simulink model "sampleModel7126_pp_1_1"  (R2018a)
settings: Solver=VariableStepAuto  StartTime=0.0  StopTime=10.0  RelTol=1e-3
undefined symbols (not defined in the file): DiscIntNeverNeededParam
libraries: simulink x367
(part 6 of 12)

== system sampleModel7126_pp_1_1/cfblk4 ==
  emi_839 : Inport
  Action Port : ActionPort  ActionType=then
  cfblk4 : simulink/Continuous/PID Controller  Controller=PID  TimeDomain=Discrete-time  SampleTime=1  IntegratorMethod=Forward Euler  FilterMethod=Forward Euler  Form=Parallel  UseFilter=on  ControllerParametersSource=internal  P=1  I=1  D=0  N=100  InitialConditionSource=internal  InitialConditionForIntegrator=0  InitialConditionForFilter=0  ExternalReset=none  LimitOutput=off  UpperSaturationLimit=inf  LowerSaturationLimit=-inf  LinearizeAsGain=off  AntiWindupMode=none  Kb=1  TrackingMode=off  Kt=1  PParamMin=[]  PParamMax=[]  IParamMin=[]  IParamMax=[]  DParamMin=[]  DParamMax=[]  NParamMin=[]  NParamMax=[]  KbParamMin=[]  KbParamMax=[]  KtParamMin=[]  KtParamMax=[]  POutMin=[]  POutMax=[]  IOutMin=[]  IOutMax=[]  DOutMin=[]  DOutMax=[]  NOutMin=[]  NOutMax=[]  KbOutMin=[]  KbOutMax=[]  KtOutMin=[]  KtOutMax=[]  IntegratorOutMin=[]  IntegratorOutMax=[]  FilterOutMin=[]  FilterOutMax=[]  SumOutMin=[]  SumOutMax=[]  SumI1OutMin=[]  SumI1OutMax=[]  SumI2OutMin=[]  SumI2OutMax=[]  SumI3OutMin=[]  SumI3OutMax=[]  SumDOutMin=[]  SumDOutMax=[]  SaturationOutMin=[]  SaturationOutMax=[]  IntegratorContinuousStateAttributes=''  IntegratorStateMustResolveToSignalObject=off  IntegratorRTWStateStorageClass=Auto  FilterContinuousStateAttributes=''  FilterStateMustResolveToSignalObject=off  FilterRTWStateStorageClass=Auto  DifferentiatorICPrevScaledInput=0  DifferentiatorOutMin=[]  DifferentiatorOutMax=[]  FilterDiffOutCoefMin=[]  FilterDiffOutCoefMax=[]  SumDenOutMin=[]  SumDenOutMax=[]  SumNumOutMin=[]  SumNumOutMax=[]  ReciprocalOutMin=[]  ReciprocalOutMax=[]  DivideOutMin=[]  DivideOutMax=[]  TunerSelectOption=Transfer Function Based (PID Tuner App)
  emi_840 : Outport
  wires:
  emi_839/1 -> cfblk4/1
  cfblk4/1 -> emi_840/1

== system sampleModel7126_pp_1_1/cfblk43 ==
  emi_1604 : Inport
  Action Port : ActionPort  ActionType=then
  cfblk43 : DiscreteFilter  SampleTime=1
  emi_1605 : Outport
  wires:
  emi_1604/1 -> cfblk43/1
  cfblk43/1 -> emi_1605/1

== system sampleModel7126_pp_1_1/cfblk44 ==
  emi_1231 : Inport
  emi_1232 : Inport  Port=2
  Action Port : ActionPort  ActionType=then
  cfblk44 : simulink/Continuous/PID Controller (2DOF)  Controller=PID  TimeDomain=Discrete-time  SampleTime=1  IntegratorMethod=Forward Euler  FilterMethod=Forward Euler  Form=Parallel  UseFilter=on  ControllerParametersSource=internal  P=1  I=1  D=0  N=100  b=1  c=1  InitialConditionSource=internal  InitialConditionForIntegrator=0  InitialConditionForFilter=0  ExternalReset=none  LimitOutput=off  UpperSaturationLimit=inf  LowerSaturationLimit=-inf  LinearizeAsGain=off  AntiWindupMode=none  Kb=1  TrackingMode=off  Kt=1  PParamMin=[]  PParamMax=[]  IParamMin=[]  IParamMax=[]  DParamMin=[]  DParamMax=[]  NParamMin=[]  NParamMax=[]  bParamMin=[]  bParamMax=[]  cParamMin=[]  cParamMax=[]  KbParamMin=[]  KbParamMax=[]  KtParamMin=[]  KtParamMax=[]  POutMin=[]  POutMax=[]  IOutMin=[]  IOutMax=[]  DOutMin=[]  DOutMax=[]  NOutMin=[]  NOutMax=[]  bOutMin=[]  bOutMax=[]  cOutMin=[]  cOutMax=[]  KbOutMin=[]  KbOutMax=[]  KtOutMin=[]  KtOutMax=[]  IntegratorOutMin=[]  IntegratorOutMax=[]  FilterOutMin=[]  FilterOutMax=[]  SumOutMin=[]  SumOutMax=[]  Sum1OutMin=[]  Sum1OutMax=[]  Sum2OutMin=[]  Sum2OutMax=[]  Sum3OutMin=[]  Sum3OutMax=[]  SumI1OutMin=[]  SumI1OutMax=[]  SumI2OutMin=[]  SumI2OutMax=[]  SumI3OutMin=[]  SumI3OutMax=[]  SumDOutMin=[]  SumDOutMax=[]  SaturationOutMin=[]  SaturationOutMax=[]  IntegratorContinuousStateAttributes=''  IntegratorStateMustResolveToSignalObject=off  IntegratorRTWStateStorageClass=Auto  FilterContinuousStateAttributes=''  FilterStateMustResolveToSignalObject=off  FilterRTWStateStorageClass=Auto  DifferentiatorICPrevScaledInput=0  DifferentiatorOutMin=[]  DifferentiatorOutMax=[]  FilterDiffOutCoefMin=[]  FilterDiffOutCoefMax=[]  SumDenOutMin=[]  SumDenOutMax=[]  SumNumOutMin=[]  SumNumOutMax=[]  ReciprocalOutMin=[]  ReciprocalOutMax=[]  DivideOutMin=[]  DivideOutMax=[]  TunerSelectOption=Transfer Function Based (PID Tuner App)
  emi_1233 : Outport
  wires:
  emi_1231/1 -> cfblk44/1
  emi_1232/1 -> cfblk44/2
  cfblk44/1 -> emi_1233/1

== system sampleModel7126_pp_1_1/cfblk48 ==
  emi_1269 : Inport
  Action Port : ActionPort  ActionType=then
  cfblk48 : DiscreteFir  SampleTime=1
  emi_1270 : Outport
  wires:
  emi_1269/1 -> cfblk48/1
  cfblk48/1 -> emi_1270/1

== system sampleModel7126_pp_1_1/cfblk5 ==
  emi_1928 : Inport
  Action Port : ActionPort  ActionType=then
  cfblk5 : DiscreteTransferFcn  SampleTime=1
  emi_1929 : Outport
  wires:
  emi_1928/1 -> cfblk5/1
  cfblk5/1 -> emi_1929/1

== system sampleModel7126_pp_1_1/cfblk54 ==
  emi_1166 : Inport
  Action Port : ActionPort  ActionType=then
  cfblk54 : simulink/Continuous/PID Controller  Controller=PID  TimeDomain=Discrete-time  SampleTime=1  IntegratorMethod=Forward Euler  FilterMethod=Forward Euler  Form=Parallel  UseFilter=on  ControllerParametersSource=internal  P=1  I=1  D=0  N=100  InitialConditionSource=internal  InitialConditionForIntegrator=0  InitialConditionForFilter=0  ExternalReset=none  LimitOutput=off  UpperSaturationLimit=inf  LowerSaturationLimit=-inf  LinearizeAsGain=off  AntiWindupMode=none  Kb=1  TrackingMode=off  Kt=1  PParamMin=[]  PParamMax=[]  IParamMin=[]  IParamMax=[]  DParamMin=[]  DParamMax=[]  NParamMin=[]  NParamMax=[]  KbParamMin=[]  KbParamMax=[]  KtParamMin=[]  KtParamMax=[]  POutMin=[]  POutMax=[]  IOutMin=[]  IOutMax=[]  DOutMin=[]  DOutMax=[]  NOutMin=[]  NOutMax=[]  KbOutMin=[]  KbOutMax=[]  KtOutMin=[]  KtOutMax=[]  IntegratorOutMin=[]  IntegratorOutMax=[]  FilterOutMin=[]  FilterOutMax=[]  SumOutMin=[]  SumOutMax=[]  SumI1OutMin=[]  SumI1OutMax=[]  SumI2OutMin=[]  SumI2OutMax=[]  SumI3OutMin=[]  SumI3OutMax=[]  SumDOutMin=[]  SumDOutMax=[]  SaturationOutMin=[]  SaturationOutMax=[]  IntegratorContinuousStateAttributes=''  IntegratorStateMustResolveToSignalObject=off  IntegratorRTWStateStorageClass=Auto  FilterContinuousStateAttributes=''  FilterStateMustResolveToSignalObject=off  FilterRTWStateStorageClass=Auto  DifferentiatorICPrevScaledInput=0  DifferentiatorOutMin=[]  DifferentiatorOutMax=[]  FilterDiffOutCoefMin=[]  FilterDiffOutCoefMax=[]  SumDenOutMin=[]  SumDenOutMax=[]  SumNumOutMin=[]  SumNumOutMax=[]  ReciprocalOutMin=[]  ReciprocalOutMax=[]  DivideOutMin=[]  DivideOutMax=[]  TunerSelectOption=Transfer Function Based (PID Tuner App)
  emi_1167 : Outport
  wires:
  emi_1166/1 -> cfblk54/1
  cfblk54/1 -> emi_1167/1

== system sampleModel7126_pp_1_1/cfblk57 ==
  emi_896 : Inport
  Action Port : ActionPort  ActionType=then
  cfblk57 : simulink/Continuous/PID Controller  Controller=PID  TimeDomain=Discrete-time  SampleTime=1  IntegratorMethod=Forward Euler  FilterMethod=Forward Euler  Form=Parallel  UseFilter=on  ControllerParametersSource=internal  P=1  I=1  D=0  N=100  InitialConditionSource=internal  InitialConditionForIntegrator=0  InitialConditionForFilter=0  ExternalReset=none  LimitOutput=off  UpperSaturationLimit=inf  LowerSaturationLimit=-inf  LinearizeAsGain=off  AntiWindupMode=none  Kb=1  TrackingMode=off  Kt=1  PParamMin=[]  PParamMax=[]  IParamMin=[]  IParamMax=[]  DParamMin=[]  DParamMax=[]  NParamMin=[]  NParamMax=[]  KbParamMin=[]  KbParamMax=[]  KtParamMin=[]  KtParamMax=[]  POutMin=[]  POutMax=[]  IOutMin=[]  IOutMax=[]  DOutMin=[]  DOutMax=[]  NOutMin=[]  NOutMax=[]  KbOutMin=[]  KbOutMax=[]  KtOutMin=[]  KtOutMax=[]  IntegratorOutMin=[]  IntegratorOutMax=[]  FilterOutMin=[]  FilterOutMax=[]  SumOutMin=[]  SumOutMax=[]  SumI1OutMin=[]  SumI1OutMax=[]  SumI2OutMin=[]  SumI2OutMax=[]  SumI3OutMin=[]  SumI3OutMax=[]  SumDOutMin=[]  SumDOutMax=[]  SaturationOutMin=[]  SaturationOutMax=[]  IntegratorContinuousStateAttributes=''  IntegratorStateMustResolveToSignalObject=off  IntegratorRTWStateStorageClass=Auto  FilterContinuousStateAttributes=''  FilterStateMustResolveToSignalObject=off  FilterRTWStateStorageClass=Auto  DifferentiatorICPrevScaledInput=0  DifferentiatorOutMin=[]  DifferentiatorOutMax=[]  FilterDiffOutCoefMin=[]  FilterDiffOutCoefMax=[]  SumDenOutMin=[]  SumDenOutMax=[]  SumNumOutMin=[]  SumNumOutMax=[]  ReciprocalOutMin=[]  ReciprocalOutMax=[]  DivideOutMin=[]  DivideOutMax=[]  TunerSelectOption=Transfer Function Based (PID Tuner App)
  emi_897 : Outport
  wires:
  emi_896/1 -> cfblk57/1
  cfblk57/1 -> emi_897/1

== system sampleModel7126_pp_1_1/cfblk60 ==
  emi_94 : Inport
  emi_95 : Inport  Port=2
  Action Port : ActionPort  ActionType=then
  cfblk60 : simulink/Continuous/PID Controller (2DOF)  Controller=PID  TimeDomain=Discrete-time  SampleTime=1  IntegratorMethod=Forward Euler  FilterMethod=Forward Euler  Form=Parallel  UseFilter=on  ControllerParametersSource=internal  P=1  I=1  D=0  N=100  b=1  c=1  InitialConditionSource=internal  InitialConditionForIntegrator=0  InitialConditionForFilter=0  ExternalReset=none  LimitOutput=off  UpperSaturationLimit=inf  LowerSaturationLimit=-inf  LinearizeAsGain=off  AntiWindupMode=none  Kb=1  TrackingMode=off  Kt=1  PParamMin=[]  PParamMax=[]  IParamMin=[]  IParamMax=[]  DParamMin=[]  DParamMax=[]  NParamMin=[]  NParamMax=[]  bParamMin=[]  bParamMax=[]  cParamMin=[]  cParamMax=[]  KbParamMin=[]  KbParamMax=[]  KtParamMin=[]  KtParamMax=[]  POutMin=[]  POutMax=[]  IOutMin=[]  IOutMax=[]  DOutMin=[]  DOutMax=[]  NOutMin=[]  NOutMax=[]  bOutMin=[]  bOutMax=[]  cOutMin=[]  cOutMax=[]  KbOutMin=[]  KbOutMax=[]  KtOutMin=[]  KtOutMax=[]  IntegratorOutMin=[]  IntegratorOutMax=[]  FilterOutMin=[]  FilterOutMax=[]  SumOutMin=[]  SumOutMax=[]  Sum1OutMin=[]  Sum1OutMax=[]  Sum2OutMin=[]  Sum2OutMax=[]  Sum3OutMin=[]  Sum3OutMax=[]  SumI1OutMin=[]  SumI1OutMax=[]  SumI2OutMin=[]  SumI2OutMax=[]  SumI3OutMin=[]  SumI3OutMax=[]  SumDOutMin=[]  SumDOutMax=[]  SaturationOutMin=[]  SaturationOutMax=[]  IntegratorContinuousStateAttributes=''  IntegratorStateMustResolveToSignalObject=off  IntegratorRTWStateStorageClass=Auto  FilterContinuousStateAttributes=''  FilterStateMustResolveToSignalObject=off  FilterRTWStateStorageClass=Auto  DifferentiatorICPrevScaledInput=0  DifferentiatorOutMin=[]  DifferentiatorOutMax=[]  FilterDiffOutCoefMin=[]  FilterDiffOutCoefMax=[]  SumDenOutMin=[]  SumDenOutMax=[]  SumNumOutMin=[]  SumNumOutMax=[]  ReciprocalOutMin=[]  ReciprocalOutMax=[]  DivideOutMin=[]  DivideOutMax=[]  TunerSelectOption=Transfer Function Based (PID Tuner App)
  emi_96 : Outport
  wires:
  emi_94/1 -> cfblk60/1
  emi_95/1 -> cfblk60/2
  cfblk60/1 -> emi_96/1

== system sampleModel7126_pp_1_1/cfblk61 ==
  emi_1138 : Inport
  Action Port : ActionPort  ActionType=then
  cfblk61 : UnitDelay
  emi_1139 : Outport
  wires:
  emi_1138/1 -> cfblk61/1
  cfblk61/1 -> emi_1139/1

== system sampleModel7126_pp_1_1/cfblk67 ==
  emi_437 : Inport
  emi_438 : Inport  Port=2
  Action Port : ActionPort  ActionType=then
  cfblk67 : Delay  ShowEnablePort=on  SampleTime=1
      settings: InputPortMap=u0,e6
  emi_439 : Outport
  wires:
  emi_437/1 -> cfblk67/1
  emi_438/1 -> cfblk67/2
  cfblk67/1 -> emi_439/1

== system sampleModel7126_pp_1_1/cfblk7 ==
  emi_1540 : Inport
  Action Port : ActionPort  ActionType=then
  cfblk7 : UnitDelay
  emi_1541 : Outport
  wires:
  emi_1540/1 -> cfblk7/1
  cfblk7/1 -> emi_1541/1

== system sampleModel7126_pp_1_1/cfblk74 ==
  emi_1569 : Inport
  Action Port : ActionPort  ActionType=then
  cfblk74 : simulink/Discrete/Tapped Delay  vinit=0.0  samptime=-1  NumDelays=1  DelayOrder=Oldest  includeCurrent=off
  emi_1570 : Outport
  wires:
  emi_1569/1 -> cfblk74/1
  cfblk74/1 -> emi_1570/1

== system sampleModel7126_pp_1_1/cfblk82 ==
  emi_2052 : Inport
  Action Port : ActionPort  ActionType=then
  cfblk82 : DiscreteTransferFcn  SampleTime=1
  emi_2053 : Outport
  wires:
  emi_2052/1 -> cfblk82/1
  cfblk82/1 -> emi_2053/1

== system sampleModel7126_pp_1_1/cfblk84 ==
  emi_2166 : Inport
  Action Port : ActionPort  ActionType=then
  cfblk84 : UnitDelay
  emi_2167 : Outport
  wires:
  emi_2166/1 -> cfblk84/1
  cfblk84/1 -> emi_2167/1

== system sampleModel7126_pp_1_1/cfblk85 ==
  emi_15 : Inport
  Action Port : ActionPort  ActionType=then
  cfblk85 : DiscreteStateSpace
  emi_16 : Outport
  wires:
  emi_15/1 -> cfblk85/1
  cfblk85/1 -> emi_16/1

== system sampleModel7126_pp_1_1/cfblk9 ==
  emi_365 : Inport
  Action Port : ActionPort  ActionType=then
  cfblk9 : DiscreteTransferFcn  SampleTime=1
  emi_366 : Outport
  wires:
  emi_365/1 -> cfblk9/1
  cfblk9/1 -> emi_366/1

== system sampleModel7126_pp_1_1/cfblk90 ==
  emi_1052 : Inport
  Action Port : ActionPort  ActionType=then
  cfblk90 : simulink/Discrete/Difference  ICPrevInput=0.0  OutMin=[]  OutMax=[]  OutDataTypeStr=double  OutputDataTypeScalingMode=double  OutDataType=fixdt(1, 16)  OutScaling=2^-10  DoSatur=off
  emi_1053 : Outport
  wires:
  emi_1052/1 -> cfblk90/1
  cfblk90/1 -> emi_1053/1

== system sampleModel7126_pp_1_1/cfblk92 ==
  emi_86 : Inport
  emi_87 : Inport  Port=2
  Action Port : ActionPort  ActionType=then
  cfblk92 : simulink/Continuous/PID Controller (2DOF)  Controller=PID  TimeDomain=Discrete-time  SampleTime=1  IntegratorMethod=Forward Euler  FilterMethod=Forward Euler  Form=Parallel  UseFilter=on  ControllerParametersSource=internal  P=1  I=1  D=0  N=100  b=1  c=1  InitialConditionSource=internal  InitialConditionForIntegrator=0  InitialConditionForFilter=0  ExternalReset=none  LimitOutput=off  UpperSaturationLimit=inf  LowerSaturationLimit=-inf  LinearizeAsGain=off  AntiWindupMode=none  Kb=1  TrackingMode=off  Kt=1  PParamMin=[]  PParamMax=[]  IParamMin=[]  IParamMax=[]  DParamMin=[]  DParamMax=[]  NParamMin=[]  NParamMax=[]  bParamMin=[]  bParamMax=[]  cParamMin=[]  cParamMax=[]  KbParamMin=[]  KbParamMax=[]  KtParamMin=[]  KtParamMax=[]  POutMin=[]  POutMax=[]  IOutMin=[]  IOutMax=[]  DOutMin=[]  DOutMax=[]  NOutMin=[]  NOutMax=[]  bOutMin=[]  bOutMax=[]  cOutMin=[]  cOutMax=[]  KbOutMin=[]  KbOutMax=[]  KtOutMin=[]  KtOutMax=[]  IntegratorOutMin=[]  IntegratorOutMax=[]  FilterOutMin=[]  FilterOutMax=[]  SumOutMin=[]  SumOutMax=[]  Sum1OutMin=[]  Sum1OutMax=[]  Sum2OutMin=[]  Sum2OutMax=[]  Sum3OutMin=[]  Sum3OutMax=[]  SumI1OutMin=[]  SumI1OutMax=[]  SumI2OutMin=[]  SumI2OutMax=[]  SumI3OutMin=[]  SumI3OutMax=[]  SumDOutMin=[]  SumDOutMax=[]  SaturationOutMin=[]  SaturationOutMax=[]  IntegratorContinuousStateAttributes=''  IntegratorStateMustResolveToSignalObject=off  IntegratorRTWStateStorageClass=Auto  FilterContinuousStateAttributes=''  FilterStateMustResolveToSignalObject=off  FilterRTWStateStorageClass=Auto  DifferentiatorICPrevScaledInput=0  DifferentiatorOutMin=[]  DifferentiatorOutMax=[]  FilterDiffOutCoefMin=[]  FilterDiffOutCoefMax=[]  SumDenOutMin=[]  SumDenOutMax=[]  SumNumOutMin=[]  SumNumOutMax=[]  ReciprocalOutMin=[]  ReciprocalOutMax=[]  DivideOutMin=[]  DivideOutMax=[]  TunerSelectOption=Transfer Function Based (PID Tuner App)
  emi_88 : Outport
  wires:
  emi_86/1 -> cfblk92/1
  emi_87/1 -> cfblk92/2
  cfblk92/1 -> emi_88/1

== system sampleModel7126_pp_1_1/cfblk97 ==
  emi_1483 : Inport
  Action Port : ActionPort  ActionType=then
  cfblk97 : simulink/Discrete/Difference  ICPrevInput=0.0  OutMin=[]  OutMax=[]  OutDataTypeStr=double  OutputDataTypeScalingMode=double  OutDataType=fixdt(1, 16)  OutScaling=2^-10  DoSatur=off
  emi_1484 : Outport
  wires:
  emi_1483/1 -> cfblk97/1
  cfblk97/1 -> emi_1484/1

== system sampleModel7126_pp_1_1/emi_1054 ==
  Action Port : ActionPort  ActionType=else
  emi_1055 : Assertion

== system sampleModel7126_pp_1_1/emi_1083 ==
  Action Port : ActionPort  ActionType=else
  emi_1084 : Assertion

== system sampleModel7126_pp_1_1/emi_1140 ==
  Action Port : ActionPort  ActionType=else
  emi_1141 : Assertion

== system sampleModel7126_pp_1_1/emi_1168 ==
  Action Port : ActionPort  ActionType=else
  emi_1169 : Assertion

== system sampleModel7126_pp_1_1/emi_1234 ==
  Action Port : ActionPort  ActionType=else
  emi_1235 : Assertion

== system sampleModel7126_pp_1_1/emi_1271 ==
  Action Port : ActionPort  ActionType=else
  emi_1272 : Assertion

== system sampleModel7126_pp_1_1/emi_1421 ==
  Action Port : ActionPort  ActionType=else
  emi_1422 : Assertion

== system sampleModel7126_pp_1_1/emi_1485 ==
  Action Port : ActionPort  ActionType=else
  emi_1486 : Assertion

== system sampleModel7126_pp_1_1/emi_1506 ==
  Action Port : ActionPort  ActionType=else
  emi_1507 : Assertion

== system sampleModel7126_pp_1_1/emi_1535 ==
  Action Port : ActionPort  ActionType=else
  emi_1536 : Assertion

== system sampleModel7126_pp_1_1/emi_1542 ==
  Action Port : ActionPort  ActionType=else
  emi_1543 : Assertion

== system sampleModel7126_pp_1_1/emi_1571 ==
  Action Port : ActionPort  ActionType=else
  emi_1572 : Assertion

== system sampleModel7126_pp_1_1/emi_1606 ==
  Action Port : ActionPort  ActionType=else
  emi_1607 : Assertion

== system sampleModel7126_pp_1_1/emi_1662 ==
  Action Port : ActionPort  ActionType=else
  emi_1663 : Assertion

== system sampleModel7126_pp_1_1/emi_17 ==
  Action Port : ActionPort  ActionType=else
  emi_18 : Assertion

== system sampleModel7126_pp_1_1/emi_1749 ==
  Action Port : ActionPort  ActionType=else
  emi_1750 : Assertion

== system sampleModel7126_pp_1_1/emi_1808 ==
  Action Port : ActionPort  ActionType=else
  emi_1809 : Assertion

== system sampleModel7126_pp_1_1/emi_1829 ==
  Action Port : ActionPort  ActionType=else
  emi_1830 : Assertion

== system sampleModel7126_pp_1_1/emi_1836 ==
  Action Port : ActionPort  ActionType=else
  emi_1837 : Assertion

== system sampleModel7126_pp_1_1/emi_189 ==
  Action Port : ActionPort  ActionType=else
  emi_190 : Assertion

== system sampleModel7126_pp_1_1/emi_1930 ==
  Action Port : ActionPort  ActionType=else
  emi_1931 : Assertion

== system sampleModel7126_pp_1_1/emi_1952 ==
  Action Port : ActionPort  ActionType=else
  emi_1953 : Assertion

== system sampleModel7126_pp_1_1/emi_197 ==
  Action Port : ActionPort  ActionType=else
  emi_198 : Assertion

== system sampleModel7126_pp_1_1/emi_2054 ==
  Action Port : ActionPort  ActionType=else
  emi_2055 : Assertion

== system sampleModel7126_pp_1_1/emi_2104 ==
  Action Port : ActionPort  ActionType=else
  emi_2105 : Assertion

== system sampleModel7126_pp_1_1/emi_2168 ==
  Action Port : ActionPort  ActionType=else
  emi_2169 : Assertion

== system sampleModel7126_pp_1_1/emi_367 ==
  Action Port : ActionPort  ActionType=else
  emi_368 : Assertion

== system sampleModel7126_pp_1_1/emi_440 ==
  Action Port : ActionPort  ActionType=else
  emi_441 : Assertion

== system sampleModel7126_pp_1_1/emi_664 ==
  Action Port : ActionPort  ActionType=else
  emi_665 : Assertion

== system sampleModel7126_pp_1_1/emi_791 ==
  Action Port : ActionPort  ActionType=else
  emi_792 : Assertion

== system sampleModel7126_pp_1_1/emi_798 ==
  Action Port : ActionPort  ActionType=else
  emi_799 : Assertion

== system sampleModel7126_pp_1_1/emi_827 ==
  Action Port : ActionPort  ActionType=else
  emi_828 : Assertion

== system sampleModel7126_pp_1_1/emi_841 ==
  Action Port : ActionPort  ActionType=else
  emi_842 : Assertion

== system sampleModel7126_pp_1_1/emi_89 ==
  Action Port : ActionPort  ActionType=else
  emi_90 : Assertion

== system sampleModel7126_pp_1_1/emi_898 ==
  Action Port : ActionPort  ActionType=else
  emi_899 : Assertion

== system sampleModel7126_pp_1_1/emi_97 ==
  Action Port : ActionPort  ActionType=else
  emi_98 : Assertion

== system sampleModel7126_pp_1_1/cfblk245/cfblk18 ==
  cfblk1 : Inport
  cfblk9 : Inport  Port=2
  Action Port : ActionPort  ActionType=then
  cfblk3 : Subsystem  TreatAsAtomicUnit=on
  cfblk4 : Delay  ShowEnablePort=on
      settings: InputPortMap=u0,e6
  cfblk5 : Subsystem  TreatAsAtomicUnit=on
  cfblk6 : simulink/Discrete/Transfer Fcn Real Zero  ZeroZ=0.75  ICPrevInput=0.0  DoSatur=off
      settings: SourceProductName=Simulink  SourceProductBaseCode=SL
  cfblk7 : Subsystem  TreatAsAtomicUnit=on
  cfblk8 : Subsystem  TreatAsAtomicUnit=on
  cyemi_{71..78} (8 alike) : DataTypeConversion  OutDataTypeStr=double
  emi_1713 : Subsystem  TreatAsAtomicUnit=on
  emi_1715 : If  IfExpression=Inf <= u1  SampleTime=[1 0]
  emi_{70,207,465,1716} (4 alike) : DataTypeConversion  OutDataTypeStr=double
  emi_204 : Subsystem  TreatAsAtomicUnit=on
  emi_206 : If  IfExpression=Inf <= u1  SampleTime=[1 0]
  emi_462 : Subsystem  TreatAsAtomicUnit=on
  emi_464 : If  IfExpression=Inf <= u1  SampleTime=[1 0]
  emi_67 : Subsystem  TreatAsAtomicUnit=on
  emi_69 : If  IfExpression=Inf <= u1
  cfblk2 : Outport
  cfblk10 : Outport  Port=2
  cfblk11 : Outport  Port=3
  wires:
  cyemi_72/1 -> cfblk4/1
  cfblk6/1 -> cyemi_72/1
  cyemi_73/1 -> cfblk4/2
  cyemi_75/1 -> cfblk6/1
  cfblk9/1 -> cyemi_75/1
  cfblk1/1 -> cyemi_76/1
  cfblk4/1 -> cyemi_77/1, cyemi_78/1, emi_70/1, emi_465/1, emi_1716/1
  cyemi_71/1 -> cfblk3/1(emi_65)
  cfblk3/1(emi_66) -> cyemi_74/1, cyemi_73/1, cfblk10/1, emi_207/1
  emi_69/1 -> cfblk3/Action
  emi_69/2 -> emi_67/Action
  emi_70/1 -> emi_69/1
  cyemi_76/1 -> cfblk7/1(emi_202)
  cfblk7/1(emi_203) -> cyemi_71/1
  emi_206/1 -> cfblk7/Action
  emi_206/2 -> emi_204/Action
  emi_207/1 -> emi_206/1
  cyemi_74/1 -> cfblk5/1(emi_460)
  cfblk5/1(emi_461) -> cfblk11/1
  emi_464/1 -> cfblk5/Action
  emi_464/2 -> emi_462/Action
  emi_465/1 -> emi_464/1
  cyemi_77/1 -> cfblk8/1(emi_1710)
  cyemi_78/1 -> cfblk8/2(emi_1711)
  cfblk8/1(emi_1712) -> cfblk2/1
  emi_1715/1 -> cfblk8/Action
  emi_1715/2 -> emi_1713/Action
  emi_1716/1 -> emi_1715/1

== system sampleModel7126_pp_1_1/cfblk245/cfblk19 ==
  cfblk1 : Inport
  Action Port : ActionPort  ActionType=else
  cfblk10 : DiscreteZeroPole  Poles=[0 0.5]  Gain=1  SampleTime=-1
  cfblk13 : Subsystem  TreatAsAtomicUnit=on
  cfblk3 : DiscreteStateSpace  SampleTime=-1
  cfblk4 : DiscreteZeroPole  Poles=[0 0.5]  Gain=1  SampleTime=-1
  cfblk5 : DiscreteZeroPole  Poles=[0 0.5]  Gain=1  SampleTime=-1
  cfblk6 : Subsystem  TreatAsAtomicUnit=on
  cfblk7 : DiscreteFir
  cfblk8 : DiscreteIntegrator  SampleTime=-1  OutDataTypeStr=double  ICPrevOutput=DiscIntNeverNeededParam  ICPrevScaledInput=DiscIntNeverNeededParam
  cfblk9 : Delay  ShowEnablePort=on
      settings: InputPortMap=u0,e6
  cyemi_{80..89} (10 alike) : DataTypeConversion  OutDataTypeStr=double
  emi_1944 : Subsystem  TreatAsAtomicUnit=on
  emi_1946 : If  IfExpression=Inf <= u1  SampleTime=[1 0]
  emi_1947 : DataTypeConversion  OutDataTypeStr=double
  emi_2161 : Subsystem  TreatAsAtomicUnit=on
  emi_2163 : If  IfExpression=Inf <= u1  SampleTime=[1 0]
  emi_2164 : DataTypeConversion  OutDataTypeStr=double
  cfblk2 : Outport
  cfblk11 : Outport  Port=2
  cfblk12 : Outport  Port=3
  wires:
  cfblk8/1 -> cyemi_85/1, cyemi_88/1, emi_1947/1
  cfblk5/1 -> cfblk11/1, cyemi_87/1, emi_2164/1
  cfblk7/1 -> cfblk12/1
  cfblk1/1 -> cfblk2/1
  cfblk4/1 -> cyemi_80/1, cyemi_89/1
  cyemi_80/1 -> cfblk10/1
  cyemi_82/1 -> cfblk3/1
  cfblk9/1 -> cyemi_82/1
  cyemi_83/1 -> cfblk4/1
  cyemi_84/1 -> cfblk5/1
  cfblk10/1 -> cyemi_84/1
  cyemi_86/1 -> cfblk7/1
  cfblk3/1 -> cyemi_86/1
  cyemi_87/1 -> cfblk8/1
  cyemi_88/1 -> cfblk9/1
  cyemi_89/1 -> cfblk9/2
  cyemi_81/1 -> cfblk13/1(emi_1942)
  cfblk13/1(emi_1943) -> cyemi_83/1
  emi_1946/1 -> cfblk13/Action
  emi_1946/2 -> emi_1944/Action
  emi_1947/1 -> emi_1946/1
  cyemi_85/1 -> cfblk6/1(emi_2159)
  cfblk6/1(emi_2160) -> cyemi_81/1
  emi_2163/1 -> cfblk6/Action
  emi_2163/2 -> emi_2161/Action
  emi_2164/1 -> emi_2163/1

== system sampleModel7126_pp_1_1/cfblk245/cfblk8 ==
  emi_669 : Inport
  Action Port : ActionPort  ActionType=then
  cfblk8 : simulink/Discrete/Tapped Delay  vinit=0.0  samptime=-1  NumDelays=1  DelayOrder=Oldest  includeCurrent=off
  emi_670 : Outport
  wires:
  emi_669/1 -> cfblk8/1
  cfblk8/1 -> emi_670/1

== system sampleModel7126_pp_1_1/cfblk245/emi_671 ==
  Action Port : ActionPort  ActionType=else
  emi_672 : Assertion

== system sampleModel7126_pp_1_1/cfblk246/cfblk10 ==
  cfblk1 : Inport
  cfblk13 : Inport  Port=2
  Action Port : ActionPort  ActionType=else
  cfblk10 : Subsystem  TreatAsAtomicUnit=on
  cfblk11 : Subsystem  TreatAsAtomicUnit=on
  cfblk12 : simulink/Continuous/PID Controller (2DOF)  Controller=PID  TimeDomain=Discrete-time  SampleTime=-1  IntegratorMethod=Forward Euler  FilterMethod=Forward Euler  Form=Parallel  UseFilter=on  ControllerParametersSource=internal  P=1  I=1  D=0  N=100  b=1  c=1  InitialConditionSource=internal  InitialConditionForIntegrator=0  InitialConditionForFilter=0  ExternalReset=none  LimitOutput=off  UpperSaturationLimit=inf  LowerSaturationLimit=-inf  LinearizeAsGain=off  AntiWindupMode=none  Kb=1  TrackingMode=off  Kt=1  PParamMin=[]  PParamMax=[]  IParamMin=[]  IParamMax=[]  DParamMin=[]  DParamMax=[]  NParamMin=[]  NParamMax=[]  bParamMin=[]  bParamMax=[]  cParamMin=[]  cParamMax=[]  KbParamMin=[]  KbParamMax=[]  KtParamMin=[]  KtParamMax=[]  POutMin=[]  POutMax=[]  IOutMin=[]  IOutMax=[]  DOutMin=[]  DOutMax=[]  NOutMin=[]  NOutMax=[]  bOutMin=[]  bOutMax=[]  cOutMin=[]  cOutMax=[]  KbOutMin=[]  KbOutMax=[]  KtOutMin=[]  KtOutMax=[]  IntegratorOutMin=[]  IntegratorOutMax=[]  FilterOutMin=[]  FilterOutMax=[]  SumOutMin=[]  SumOutMax=[]  Sum1OutMin=[]  Sum1OutMax=[]  Sum2OutMin=[]  Sum2OutMax=[]  Sum3OutMin=[]  Sum3OutMax=[]  SumI1OutMin=[]  SumI1OutMax=[]  SumI2OutMin=[]  SumI2OutMax=[]  SumI3OutMin=[]  SumI3OutMax=[]  SumDOutMin=[]  SumDOutMax=[]  SaturationOutMin=[]  SaturationOutMax=[]  IntegratorContinuousStateAttributes=''  IntegratorStateMustResolveToSignalObject=off  IntegratorRTWStateStorageClass=Auto  FilterContinuousStateAttributes=''  FilterStateMustResolveToSignalObject=off  FilterRTWStateStorageClass=Auto  DifferentiatorICPrevScaledInput=0  DifferentiatorOutMin=[]  DifferentiatorOutMax=[]  FilterDiffOutCoefMin=[]  FilterDiffOutCoefMax=[]  SumDenOutMin=[]  SumDenOutMax=[]  SumNumOutMin=[]  SumNumOutMax=[]  ReciprocalOutMin=[]  ReciprocalOutMax=[]  DivideOutMin=[]  DivideOutMax=[]  TunerSelectOption=Transfer Function Based (PID Tuner App)
  cfblk16 : Subsystem  TreatAsAtomicUnit=on
  cfblk17 : Delay
  cfblk3 : Subsystem  TreatAsAtomicUnit=on
  cfblk4 : DiscreteZeroPole  Poles=[0 0.5]  Gain=1  SampleTime=-1
  cfblk5 : Delay  DelayLengthSource=Input port
      settings: InputPortMap=u0,p1
  cfblk6 : Delay  DelayLengthSource=Input port
      settings: InputPortMap=u0,p1
  cfblk7 : simulink/Continuous/PID Controller  Controller=PID  TimeDomain=Discrete-time  SampleTime=-1  IntegratorMethod=Forward Euler  FilterMethod=Forward Euler  Form=Parallel  UseFilter=on  ControllerParametersSource=internal  P=1  I=1  D=0  N=100  InitialConditionSource=internal  InitialConditionForIntegrator=0  InitialConditionForFilter=0  ExternalReset=none  LimitOutput=off  UpperSaturationLimit=inf  LowerSaturationLimit=-inf  LinearizeAsGain=off  AntiWindupMode=none  Kb=1  TrackingMode=off  Kt=1  PParamMin=[]  PParamMax=[]  IParamMin=[]  IParamMax=[]  DParamMin=[]  DParamMax=[]  NParamMin=[]  NParamMax=[]  KbParamMin=[]  KbParamMax=[]  KtParamMin=[]  KtParamMax=[]  POutMin=[]  POutMax=[]  IOutMin=[]  IOutMax=[]  DOutMin=[]  DOutMax=[]  NOutMin=[]  NOutMax=[]  KbOutMin=[]  KbOutMax=[]  KtOutMin=[]  KtOutMax=[]  IntegratorOutMin=[]  IntegratorOutMax=[]  FilterOutMin=[]  FilterOutMax=[]  SumOutMin=[]  SumOutMax=[]  SumI1OutMin=[]  SumI1OutMax=[]  SumI2OutMin=[]  SumI2OutMax=[]  SumI3OutMin=[]  SumI3OutMax=[]  SumDOutMin=[]  SumDOutMax=[]  SaturationOutMin=[]  SaturationOutMax=[]  IntegratorContinuousStateAttributes=''  IntegratorStateMustResolveToSignalObject=off  IntegratorRTWStateStorageClass=Auto  FilterContinuousStateAttributes=''  FilterStateMustResolveToSignalObject=off  FilterRTWStateStorageClass=Auto  DifferentiatorICPrevScaledInput=0  DifferentiatorOutMin=[]  DifferentiatorOutMax=[]  FilterDiffOutCoefMin=[]  FilterDiffOutCoefMax=[]  SumDenOutMin=[]  SumDenOutMax=[]  SumNumOutMin=[]  SumNumOutMax=[]  ReciprocalOutMin=[]  ReciprocalOutMax=[]  DivideOutMin=[]  DivideOutMax=[]  TunerSelectOption=Transfer Function Based (PID Tuner App)
  cfblk8 : DiscreteZeroPole  Poles=[0 0.5]  Gain=1  SampleTime=-1
  cfblk9 : DiscreteFir
  cyemi_{103..117} (15 alike) : DataTypeConversion  OutDataTypeStr=double
  emi_154 : Subsystem  TreatAsAtomicUnit=on
  emi_156 : If  IfExpression=0 <= u1
  emi_{157,320,596,2135} (4 alike) : DataTypeConversion  OutDataTypeStr=double
  emi_2132 : Subsystem  TreatAsAtomicUnit=on
  emi_2134 : If  IfExpression=0 <= u1  SampleTime=[1 0]
  emi_317 : Subsystem  TreatAsAtomicUnit=on
  emi_319 : If  IfExpression=0 <= u1  SampleTime=[1 0]
  emi_593 : Subsystem  TreatAsAtomicUnit=on
  emi_595 : If  IfExpression=0 <= u1  SampleTime=[1 0]
  cfblk2 : Outport
  cfblk14 : Outport  Port=2
  cfblk15 : Outport  Port=3
  wires:
  cfblk9/1 -> cyemi_103/1, cyemi_108/1, emi_157/1
  cfblk5/1 -> cfblk14/1, cfblk2/1
  cfblk6/1 -> cyemi_104/1, cyemi_112/1
  cfblk8/1 -> cfblk15/1, cyemi_114/1, emi_596/1, emi_2135/1
  cyemi_105/1 -> cfblk12/1
  cyemi_106/1 -> cfblk12/2
  cfblk17/1 -> cyemi_106/1
  cyemi_108/1 -> cfblk17/1
  cyemi_110/1 -> cfblk4/1
  cfblk12/1 -> cyemi_110/1
  cyemi_111/1 -> cfblk5/1
  cfblk13/1 -> cyemi_111/1
  cyemi_112/1 -> cfblk5/2
  cyemi_113/1 -> cfblk6/1
  cyemi_114/1 -> cfblk6/2
  cyemi_115/1 -> cfblk7/1
  cfblk1/1 -> cyemi_115/1
  cyemi_116/1 -> cfblk8/1
  cfblk7/1 -> cyemi_116/1
  cyemi_117/1 -> cfblk9/1
  cfblk4/1 -> cyemi_117/1, emi_320/1
  cyemi_103/1 -> cfblk10/1(emi_152)
  cfblk10/1(emi_153) -> cyemi_109/1
  emi_156/1 -> cfblk10/Action
  emi_156/2 -> emi_154/Action
  emi_157/1 -> emi_156/1
  cyemi_107/1 -> cfblk16/1(emi_315)
  cfblk16/1(emi_316) -> cyemi_113/1
  emi_319/1 -> cfblk16/Action
  emi_319/2 -> emi_317/Action
  emi_320/1 -> emi_319/1
  cyemi_104/1 -> cfblk11/1(emi_591)
  cfblk11/1(emi_592) -> cyemi_105/1
  emi_595/1 -> cfblk11/Action
  emi_595/2 -> emi_593/Action
  emi_596/1 -> emi_595/1
  cyemi_109/1 -> cfblk3/1(emi_2130)
  cfblk3/1(emi_2131) -> cyemi_107/1
  emi_2134/1 -> cfblk3/Action
  emi_2134/2 -> emi_2132/Action
  emi_2135/1 -> emi_2134/1

== system sampleModel7126_pp_1_1/cfblk246/cfblk4 ==
  emi_513 : Inport
  Action Port : ActionPort  ActionType=then
  cfblk4 : DiscreteStateSpace  SampleTime=-1
  emi_514 : Outport
  wires:
  emi_513/1 -> cfblk4/1
  cfblk4/1 -> emi_514/1

== system sampleModel7126_pp_1_1/cfblk246/cfblk5 ==
  emi_1862 : Inport
  Action Port : ActionPort  ActionType=then
  cfblk5 : simulink/Discrete/Transfer Fcn Lead or Lag  PoleZ=0.95  ZeroZ=0.75  ICPrevOutput=0.0  ICPrevInput=0.0  DoSatur=off
      settings: SourceProductName=Simulink  SourceProductBaseCode=SL
  emi_1863 : Outport
  wires:
  emi_1862/1 -> cfblk5/1
  cfblk5/1 -> emi_1863/1

== system sampleModel7126_pp_1_1/cfblk246/cfblk9 ==
  cfblk1 : Inport
  Action Port : ActionPort  ActionType=then
  cfblk10 : simulink/Discrete/Difference  ICPrevInput=0.0  OutMin=[]  OutMax=[]  OutDataTypeStr=double  OutputDataTypeScalingMode=double  OutDataType=fixdt(1, 16)  OutScaling=2^-10  DoSatur=off
  cfblk3 : Delay
  cfblk4 : simulink/Discrete/Tapped Delay  vinit=0.0  samptime=-1  NumDelays=1  DelayOrder=Oldest  includeCurrent=off
  cfblk5 : simulink/Discrete/Difference  ICPrevInput=0.0  OutMin=[]  OutMax=[]  OutDataTypeStr=double  OutputDataTypeScalingMode=double  OutDataType=fixdt(1, 16)  OutScaling=2^-10  DoSatur=off
  cfblk6 : simulink/Discrete/Transfer Fcn Lead or Lag  PoleZ=0.95  ZeroZ=0.75  ICPrevOutput=0.0  ICPrevInput=0.0  DoSatur=off
      settings: SourceProductName=Simulink  SourceProductBaseCode=SL
  cfblk7 : Subsystem  TreatAsAtomicUnit=on
  cfblk8 : simulink/Discrete/Difference  ICPrevInput=0.0  OutMin=[]  OutMax=[]  OutDataTypeStr=double  OutputDataTypeScalingMode=double  OutDataType=fixdt(1, 16)  OutScaling=2^-10  DoSatur=off
  cfblk9 : UnitDelay  SampleTime=-1
  cyemi_{125..132} (8 alike) : DataTypeConversion  OutDataTypeStr=double
  emi_1901 : Subsystem  TreatAsAtomicUnit=on
  emi_1903 : If  IfExpression=0 <= u1  SampleTime=[1 0]
  emi_1904 : DataTypeConversion  OutDataTypeStr=double
  cfblk2 : Outport
  cfblk11 : Outport  Port=2
  wires:
  cfblk8/1 -> cfblk2/1
  cfblk9/1 -> cyemi_125/1, cyemi_130/1
  cfblk3/1 -> cfblk11/1, emi_1904/1
  cyemi_125/1 -> cfblk10/1
  cyemi_126/1 -> cfblk3/1
  cfblk10/1 -> cyemi_126/1
  cyemi_127/1 -> cfblk4/1
  cfblk6/1 -> cyemi_127/1
  cyemi_128/1 -> cfblk5/1
  cfblk4/1 -> cyemi_128/1
  cyemi_129/1 -> cfblk6/1
  cyemi_131/1 -> cfblk8/1
  cfblk5/1 -> cyemi_131/1
  cyemi_132/1 -> cfblk9/1
  cfblk1/1 -> cyemi_132/1
  cyemi_130/1 -> cfblk7/1(emi_1899)
  cfblk7/1(emi_1900) -> cyemi_129/1
  emi_1903/1 -> cfblk7/Action
  emi_1903/2 -> emi_1901/Action
  emi_1904/1 -> emi_1903/1

== system sampleModel7126_pp_1_1/cfblk246/emi_1864 ==
  Action Port : ActionPort  ActionType=else
  emi_1865 : Assertion

== system sampleModel7126_pp_1_1/cfblk246/emi_515 ==
  Action Port : ActionPort  ActionType=else
  emi_516 : Assertion

== system sampleModel7126_pp_1_1/cfblk247/cfblk18 ==
  cfblk1 : Inport
  cfblk11 : Inport  Port=2
  cfblk12 : Inport  Port=3
  cfblk13 : Inport  Port=4
  Action Port : ActionPort  ActionType=then
  cfblk10 : DiscreteStateSpace  SampleTime=-1
  cfblk17 : Delay
  cfblk3 : DiscreteZeroPole  Poles=[0 0.5]  Gain=1  SampleTime=-1
  cfblk4 : DiscreteZeroPole  Poles=[0 0.5]  Gain=1  SampleTime=-1
  cfblk5 : simulink/Discrete/Difference  ICPrevInput=0.0  OutMin=[]  OutMax=[]  OutDataTypeStr=double  OutputDataTypeScalingMode=double  OutDataType=fixdt(1, 16)  OutScaling=2^-10  DoSatur=off
  cfblk6 : simulink/Discrete/Transfer Fcn Lead or Lag  PoleZ=0.95  ZeroZ=0.75  ICPrevOutput=0.0  ICPrevInput=0.0  DoSatur=off
      settings: SourceProductName=Simulink  SourceProductBaseCode=SL
  cfblk7 : DiscreteFilter
  cfblk8 : Delay  ShowEnablePort=on
      settings: InputPortMap=u0,e6
  cfblk9 : Subsystem  TreatAsAtomicUnit=on
  cyemi_{145..154} (10 alike) : DataTypeConversion  OutDataTypeStr=double
  emi_1987 : Subsystem  TreatAsAtomicUnit=on
  emi_1989 : If  IfExpression=Inf <= u1  SampleTime=[1 0]
  emi_1990 : DataTypeConversion  OutDataTypeStr=double
  cfblk2 : Outport
  cfblk14 : Outport  Port=2
  cfblk15 : Outport  Port=3
  cfblk16 : Outport  Port=4
  wires:
  cfblk3/1 -> cfblk16/1, emi_1990/1
  cfblk13/1 -> cfblk14/1
  cfblk10/1 -> cfblk15/1
  cfblk6/1 -> cyemi_145/1, cyemi_149/1
  cfblk1/1 -> cfblk2/1
  cyemi_145/1 -> cfblk10/1
  cyemi_146/1 -> cfblk17/1
  cfblk7/1 -> cyemi_146/1
  cyemi_147/1 -> cfblk3/1
  cfblk11/1 -> cyemi_147/1
  cyemi_148/1 -> cfblk4/1
  cfblk5/1 -> cyemi_148/1
  cyemi_149/1 -> cfblk5/1
  cyemi_150/1 -> cfblk6/1
  cfblk12/1 -> cyemi_150/1
  cyemi_151/1 -> cfblk7/1
  cyemi_152/1 -> cfblk8/1
  cfblk17/1 -> cyemi_152/1
  cyemi_153/1 -> cfblk8/2
  cfblk4/1 -> cyemi_153/1
  cfblk8/1 -> cyemi_154/1
  cyemi_154/1 -> cfblk9/1(emi_1985)
  cfblk9/1(emi_1986) -> cyemi_151/1
  emi_1989/1 -> cfblk9/Action
  emi_1989/2 -> emi_1987/Action
  emi_1990/1 -> emi_1989/1

== system sampleModel7126_pp_1_1/cfblk247/cfblk19 ==
  cfblk1 : Inport
  cfblk11 : Inport  Port=2
  Action Port : ActionPort  ActionType=else
  cfblk10 : Subsystem  TreatAsAtomicUnit=on
  cfblk14 : Subsystem  TreatAsAtomicUnit=on
  cfblk3 : DiscreteFilter
  cfblk4 : simulink/Discrete/Tapped Delay  vinit=0.0  samptime=-1  NumDelays=1  DelayOrder=Oldest  includeCurrent=off
  cfblk5 : simulink/Discrete/Transfer Fcn First Order  PoleZ=0.95  ICPrevOutput=0.0  DoSatur=off
      settings: SourceProductName=Simulink
  cfblk6 : simulink/Discrete/Transfer Fcn Real Zero  ZeroZ=0.75  ICPrevInput=0.0  DoSatur=off
      settings: SourceProductName=Simulink  SourceProductBaseCode=SL
  cfblk7 : simulink/Continuous/PID Controller  Controller=PID  TimeDomain=Discrete-time  SampleTime=-1  IntegratorMethod=Forward Euler  FilterMethod=Forward Euler  Form=Parallel  UseFilter=on  ControllerParametersSource=internal  P=1  I=1  D=0  N=100  InitialConditionSource=internal  InitialConditionForIntegrator=0  InitialConditionForFilter=0  ExternalReset=none  LimitOutput=off  UpperSaturationLimit=inf  LowerSaturationLimit=-inf  LinearizeAsGain=off  AntiWindupMode=none  Kb=1  TrackingMode=off  Kt=1  PParamMin=[]  PParamMax=[]  IParamMin=[]  IParamMax=[]  DParamMin=[]  DParamMax=[]  NParamMin=[]  NParamMax=[]  KbParamMin=[]  KbParamMax=[]  KtParamMin=[]  KtParamMax=[]  POutMin=[]  POutMax=[]  IOutMin=[]  IOutMax=[]  DOutMin=[]  DOutMax=[]  NOutMin=[]  NOutMax=[]  KbOutMin=[]  KbOutMax=[]  KtOutMin=[]  KtOutMax=[]  IntegratorOutMin=[]  IntegratorOutMax=[]  FilterOutMin=[]  FilterOutMax=[]  SumOutMin=[]  SumOutMax=[]  SumI1OutMin=[]  SumI1OutMax=[]  SumI2OutMin=[]  SumI2OutMax=[]  SumI3OutMin=[]  SumI3OutMax=[]  SumDOutMin=[]  SumDOutMax=[]  SaturationOutMin=[]  SaturationOutMax=[]  IntegratorContinuousStateAttributes=''  IntegratorStateMustResolveToSignalObject=off  IntegratorRTWStateStorageClass=Auto  FilterContinuousStateAttributes=''  FilterStateMustResolveToSignalObject=off  FilterRTWStateStorageClass=Auto  DifferentiatorICPrevScaledInput=0  DifferentiatorOutMin=[]  DifferentiatorOutMax=[]  FilterDiffOutCoefMin=[]  FilterDiffOutCoefMax=[]  SumDenOutMin=[]  SumDenOutMax=[]  SumNumOutMin=[]  SumNumOutMax=[]  ReciprocalOutMin=[]  ReciprocalOutMax=[]  DivideOutMin=[]  DivideOutMax=[]  TunerSelectOption=Transfer Function Based (PID Tuner App)
  cfblk8 : UnitDelay  SampleTime=-1
  cfblk9 : simulink/Discrete/Transfer Fcn First Order  PoleZ=0.95  ICPrevOutput=0.0  DoSatur=off
      settings: SourceProductName=Simulink
  cyemi_{157..165} (9 alike) : DataTypeConversion  OutDataTypeStr=double
  emi_1026 : Subsystem  TreatAsAtomicUnit=on
  emi_1028 : If  IfExpression=0 <= u1
  emi_1029 : DataTypeConversion  OutDataTypeStr=double
  emi_282 : Subsystem  TreatAsAtomicUnit=on
  emi_284 : If  IfExpression=0 <= u1  SampleTime=[1 0]
  emi_285 : DataTypeConversion  OutDataTypeStr=double
  cfblk2 : Outport
  cfblk12 : Outport  Port=2
  cfblk13 : Outport  Port=3
  wires:
  cfblk3/1 -> cfblk12/1
  cfblk7/1 -> cfblk2/1
  cfblk8/1 -> cfblk13/1
  cfblk11/1 -> cyemi_161/1, cyemi_164/1
  cfblk5/1 -> cyemi_157/1
  cfblk6/1 -> cyemi_158/1
  cyemi_159/1 -> cfblk3/1
  cfblk1/1 -> cyemi_159/1
  cyemi_160/1 -> cfblk4/1
  cyemi_161/1 -> cfblk5/1
  cyemi_162/1 -> cfblk6/1
  cfblk4/1 -> cyemi_162/1, emi_285/1
  cyemi_163/1 -> cfblk7/1
  cfblk9/1 -> cyemi_163/1
  cyemi_164/1 -> cfblk8/1
  cyemi_165/1 -> cfblk9/1
  cyemi_158/1 -> cfblk14/1(emi_280)
  cfblk14/1(emi_281) -> cyemi_160/1, emi_1029/1
  emi_284/1 -> cfblk14/Action
  emi_284/2 -> emi_282/Action
  emi_285/1 -> emi_284/1
  cyemi_157/1 -> cfblk10/1(emi_1024)
  cfblk10/1(emi_1025) -> cyemi_165/1
  emi_1028/1 -> cfblk10/Action
  emi_1028/2 -> emi_1026/Action
  emi_1029/1 -> emi_1028/1

== system sampleModel7126_pp_1_1/cfblk247/cfblk23 ==
  emi_619 : Inport
  Action Port : ActionPort  ActionType=then
  cfblk23 : Delay
  emi_620 : Outport
  wires:
  emi_619/1 -> cfblk23/1
  cfblk23/1 -> emi_620/1

== system sampleModel7126_pp_1_1/cfblk247/cfblk3 ==
  emi_1180 : Inport
  emi_1181 : Inport  Port=2
  Action Port : ActionPort  ActionType=then
  cfblk3 : Delay  ShowEnablePort=on
      settings: InputPortMap=u0,e6
  emi_1182 : Outport
  wires:
  emi_1180/1 -> cfblk3/1
  emi_1181/1 -> cfblk3/2
  cfblk3/1 -> emi_1182/1

== system sampleModel7126_pp_1_1/cfblk247/cfblk4 ==
  emi_497 : Inport
  emi_498 : Inport  Port=2
  Action Port : ActionPort  ActionType=then
  cfblk4 : simulink/Continuous/PID Controller (2DOF)  Controller=PID  TimeDomain=Discrete-time  SampleTime=-1  IntegratorMethod=Forward Euler  FilterMethod=Forward Euler  Form=Parallel  UseFilter=on  ControllerParametersSource=internal  P=1  I=1  D=0  N=100  b=1  c=1  InitialConditionSource=internal  InitialConditionForIntegrator=0  InitialConditionForFilter=0  ExternalReset=none  LimitOutput=off  UpperSaturationLimit=inf  LowerSaturationLimit=-inf  LinearizeAsGain=off  AntiWindupMode=none  Kb=1  TrackingMode=off  Kt=1  PParamMin=[]  PParamMax=[]  IParamMin=[]  IParamMax=[]  DParamMin=[]  DParamMax=[]  NParamMin=[]  NParamMax=[]  bParamMin=[]  bParamMax=[]  cParamMin=[]  cParamMax=[]  KbParamMin=[]  KbParamMax=[]  KtParamMin=[]  KtParamMax=[]  POutMin=[]  POutMax=[]  IOutMin=[]  IOutMax=[]  DOutMin=[]  DOutMax=[]  NOutMin=[]  NOutMax=[]  bOutMin=[]  bOutMax=[]  cOutMin=[]  cOutMax=[]  KbOutMin=[]  KbOutMax=[]  KtOutMin=[]  KtOutMax=[]  IntegratorOutMin=[]  IntegratorOutMax=[]  FilterOutMin=[]  FilterOutMax=[]  SumOutMin=[]  SumOutMax=[]  Sum1OutMin=[]  Sum1OutMax=[]  Sum2OutMin=[]  Sum2OutMax=[]  Sum3OutMin=[]  Sum3OutMax=[]  SumI1OutMin=[]  SumI1OutMax=[]  SumI2OutMin=[]  SumI2OutMax=[]  SumI3OutMin=[]  SumI3OutMax=[]  SumDOutMin=[]  SumDOutMax=[]  SaturationOutMin=[]  SaturationOutMax=[]  IntegratorContinuousStateAttributes=''  IntegratorStateMustResolveToSignalObject=off  IntegratorRTWStateStorageClass=Auto  FilterContinuousStateAttributes=''  FilterStateMustResolveToSignalObject=off  FilterRTWStateStorageClass=Auto  DifferentiatorICPrevScaledInput=0  DifferentiatorOutMin=[]  DifferentiatorOutMax=[]  FilterDiffOutCoefMin=[]  FilterDiffOutCoefMax=[]  SumDenOutMin=[]  SumDenOutMax=[]  SumNumOutMin=[]  SumNumOutMax=[]  ReciprocalOutMin=[]  ReciprocalOutMax=[]  DivideOutMin=[]  DivideOutMax=[]  TunerSelectOption=Transfer Function Based (PID Tuner App)
  emi_499 : Outport
  wires:
  emi_497/1 -> cfblk4/1
  emi_498/1 -> cfblk4/2
  cfblk4/1 -> emi_499/1

== system sampleModel7126_pp_1_1/cfblk247/emi_1183 ==
  Action Port : ActionPort  ActionType=else
  emi_1184 : Assertion

== system sampleModel7126_pp_1_1/cfblk247/emi_500 ==
  Action Port : ActionPort  ActionType=else
  emi_501 : Assertion

== system sampleModel7126_pp_1_1/cfblk247/emi_621 ==
  Action Port : ActionPort  ActionType=else
  emi_622 : Assertion

== system sampleModel7126_pp_1_1/cfblk248/cfblk10 ==
  emi_102 : Inport
  Action Port : ActionPort  ActionType=then
  cfblk10 : DiscreteFilter
  emi_103 : Outport
  wires:
  emi_102/1 -> cfblk10/1
  cfblk10/1 -> emi_103/1

== system sampleModel7126_pp_1_1/cfblk248/cfblk13 ==
  emi_2037 : Inport
  emi_2038 : Inport  Port=2
  Action Port : ActionPort  ActionType=then
  cfblk13 : Delay  ShowEnablePort=on
      settings: InputPortMap=u0,e6
  emi_2039 : Outport
  wires:
  emi_2037/1 -> cfblk13/1
  emi_2038/1 -> cfblk13/2
  cfblk13/1 -> emi_2039/1

== system sampleModel7126_pp_1_1/cfblk248/cfblk14 ==
  emi_967 : Inport
  Action Port : ActionPort  ActionType=then
  cfblk14 : simulink/Discrete/Transfer Fcn Real Zero  ZeroZ=0.75  ICPrevInput=0.0  DoSatur=off
      settings: SourceProductName=Simulink  SourceProductBaseCode=SL
  emi_968 : Outport
  wires:
  emi_967/1 -> cfblk14/1
  cfblk14/1 -> emi_968/1

== system sampleModel7126_pp_1_1/cfblk248/cfblk20 ==
  emi_337 : Inport
  Action Port : ActionPort  ActionType=then
  cfblk20 : DataTypeConversion  OutDataTypeStr=double
  emi_338 : Outport
  wires:
  emi_337/1 -> cfblk20/1
  cfblk20/1 -> emi_338/1

== system sampleModel7126_pp_1_1/cfblk248/cfblk21 ==
  emi_1576 : Inport
  Action Port : ActionPort  ActionType=then
  cfblk21 : DataTypeConversion  OutDataTypeStr=uint32
  emi_1577 : Outport
  wires:
  emi_1576/1 -> cfblk21/1
  cfblk21/1 -> emi_1577/1

== system sampleModel7126_pp_1_1/cfblk248/cfblk3 ==
  emi_1476 : Inport
  Action Port : ActionPort  ActionType=then
  cfblk3 : DiscreteFir
  emi_1477 : Outport
  wires:
  emi_1476/1 -> cfblk3/1
  cfblk3/1 -> emi_1477/1

== system sampleModel7126_pp_1_1/cfblk248/cfblk5 ==
  emi_386 : Inport
  Action Port : ActionPort  ActionType=then
  cfblk5 : DiscreteZeroPole  Poles=[0 0.5]  Gain=1  SampleTime=-1
  emi_387 : Outport
  wires:
  emi_386/1 -> cfblk5/1
  cfblk5/1 -> emi_387/1

== system sampleModel7126_pp_1_1/cfblk248/cfblk6 ==
  emi_697 : Inport
  Action Port : ActionPort  ActionType=then
  cfblk6 : simulink/Continuous/PID Controller  Controller=PID  TimeDomain=Discrete-time  SampleTime=-1  IntegratorMethod=Forward Euler  FilterMethod=Forward Euler  Form=Parallel  UseFilter=on  ControllerParametersSource=internal  P=1  I=1  D=0  N=100  InitialConditionSource=internal  InitialConditionForIntegrator=0  InitialConditionForFilter=0  ExternalReset=none  LimitOutput=off  UpperSaturationLimit=inf  LowerSaturationLimit=-inf  LinearizeAsGain=off  AntiWindupMode=none  Kb=1  TrackingMode=off  Kt=1  PParamMin=[]  PParamMax=[]  IParamMin=[]  IParamMax=[]  DParamMin=[]  DParamMax=[]  NParamMin=[]  NParamMax=[]  KbParamMin=[]  KbParamMax=[]  KtParamMin=[]  KtParamMax=[]  POutMin=[]  POutMax=[]  IOutMin=[]  IOutMax=[]  DOutMin=[]  DOutMax=[]  NOutMin=[]  NOutMax=[]  KbOutMin=[]  KbOutMax=[]  KtOutMin=[]  KtOutMax=[]  IntegratorOutMin=[]  IntegratorOutMax=[]  FilterOutMin=[]  FilterOutMax=[]  SumOutMin=[]  SumOutMax=[]  SumI1OutMin=[]  SumI1OutMax=[]  SumI2OutMin=[]  SumI2OutMax=[]  SumI3OutMin=[]  SumI3OutMax=[]  SumDOutMin=[]  SumDOutMax=[]  SaturationOutMin=[]  SaturationOutMax=[]  IntegratorContinuousStateAttributes=''  IntegratorStateMustResolveToSignalObject=off  IntegratorRTWStateStorageClass=Auto  FilterContinuousStateAttributes=''  FilterStateMustResolveToSignalObject=off  FilterRTWStateStorageClass=Auto  DifferentiatorICPrevScaledInput=0  DifferentiatorOutMin=[]  DifferentiatorOutMax=[]  FilterDiffOutCoefMin=[]  FilterDiffOutCoefMax=[]  SumDenOutMin=[]  SumDenOutMax=[]  SumNumOutMin=[]  SumNumOutMax=[]  ReciprocalOutMin=[]  ReciprocalOutMax=[]  DivideOutMin=[]  DivideOutMax=[]  TunerSelectOption=Transfer Function Based (PID Tuner App)
  emi_698 : Outport
  wires:
  emi_697/1 -> cfblk6/1
  cfblk6/1 -> emi_698/1

== system sampleModel7126_pp_1_1/cfblk248/cfblk7 ==
  emi_2014 : Inport
  emi_2015 : Inport  Port=2
  Action Port : ActionPort  ActionType=then
  cfblk7 : simulink/Continuous/PID Controller (2DOF)  Controller=PID  TimeDomain=Discrete-time  SampleTime=-1  IntegratorMethod=Forward Euler  FilterMethod=Forward Euler  Form=Parallel  UseFilter=on  ControllerParametersSource=internal  P=1  I=1  D=0  N=100  b=1  c=1  InitialConditionSource=internal  InitialConditionForIntegrator=0  InitialConditionForFilter=0  ExternalReset=none  LimitOutput=off  UpperSaturationLimit=inf  LowerSaturationLimit=-inf  LinearizeAsGain=off  AntiWindupMode=none  Kb=1  TrackingMode=off  Kt=1  PParamMin=[]  PParamMax=[]  IParamMin=[]  IParamMax=[]  DParamMin=[]  DParamMax=[]  NParamMin=[]  NParamMax=[]  bParamMin=[]  bParamMax=[]  cParamMin=[]  cParamMax=[]  KbParamMin=[]  KbParamMax=[]  KtParamMin=[]  KtParamMax=[]  POutMin=[]  POutMax=[]  IOutMin=[]  IOutMax=[]  DOutMin=[]  DOutMax=[]  NOutMin=[]  NOutMax=[]  bOutMin=[]  bOutMax=[]  cOutMin=[]  cOutMax=[]  KbOutMin=[]  KbOutMax=[]  KtOutMin=[]  KtOutMax=[]  IntegratorOutMin=[]  IntegratorOutMax=[]  FilterOutMin=[]  FilterOutMax=[]  SumOutMin=[]  SumOutMax=[]  Sum1OutMin=[]  Sum1OutMax=[]  Sum2OutMin=[]  Sum2OutMax=[]  Sum3OutMin=[]  Sum3OutMax=[]  SumI1OutMin=[]  SumI1OutMax=[]  SumI2OutMin=[]  SumI2OutMax=[]  SumI3OutMin=[]  SumI3OutMax=[]  SumDOutMin=[]  SumDOutMax=[]  SaturationOutMin=[]  SaturationOutMax=[]  IntegratorContinuousStateAttributes=''  IntegratorStateMustResolveToSignalObject=off  IntegratorRTWStateStorageClass=Auto  FilterContinuousStateAttributes=''  FilterStateMustResolveToSignalObject=off  FilterRTWStateStorageClass=Auto  DifferentiatorICPrevScaledInput=0  DifferentiatorOutMin=[]  DifferentiatorOutMax=[]  FilterDiffOutCoefMin=[]  FilterDiffOutCoefMax=[]  SumDenOutMin=[]  SumDenOutMax=[]  SumNumOutMin=[]  SumNumOutMax=[]  ReciprocalOutMin=[]  ReciprocalOutMax=[]  DivideOutMin=[]  DivideOutMax=[]  TunerSelectOption=Transfer Function Based (PID Tuner App)
  emi_2016 : Outport
  wires:
  emi_2014/1 -> cfblk7/1
  emi_2015/1 -> cfblk7/2
  cfblk7/1 -> emi_2016/1

== system sampleModel7126_pp_1_1/cfblk248/emi_104 ==
  Action Port : ActionPort  ActionType=else
  emi_105 : Assertion

== system sampleModel7126_pp_1_1/cfblk248/emi_1478 ==
  Action Port : ActionPort  ActionType=else
  emi_1479 : Assertion

== system sampleModel7126_pp_1_1/cfblk248/emi_1578 ==
  Action Port : ActionPort  ActionType=else
  emi_1579 : Assertion

== system sampleModel7126_pp_1_1/cfblk248/emi_2017 ==
  Action Port : ActionPort  ActionType=else
  emi_2018 : Assertion

== system sampleModel7126_pp_1_1/cfblk248/emi_2040 ==
  Action Port : ActionPort  ActionType=else
  emi_2041 : Assertion

== system sampleModel7126_pp_1_1/cfblk248/emi_339 ==
  Action Port : ActionPort  ActionType=else
  emi_340 : Assertion

== system sampleModel7126_pp_1_1/cfblk248/emi_388 ==
  Action Port : ActionPort  ActionType=else
  emi_389 : Assertion

== system sampleModel7126_pp_1_1/cfblk248/emi_699 ==
  Action Port : ActionPort  ActionType=else
  emi_700 : Assertion

== system sampleModel7126_pp_1_1/cfblk248/emi_969 ==
  Action Port : ActionPort  ActionType=else
  emi_970 : Assertion
